simulink model "Control_Sim"  (R2023b)
settings: Solver=ode4  StartTime=0.0  StopTime=tf  FixedStep=tstep  RelTol=1e-3  EnableMultiTasking=on
values from neighbouring files (symbols this model uses):
  A_ref = [0 1;          -2*zeta*w_n_p -w_n_p^2]    [Velocity_Control.m]
  B_ref = [0; 1]    [Velocity_Control.m]
  count_map = zeros(length(theta),length(phi))    [Velocity_Control.m]
  g = 9.8065    [Velocity_Control.m]
  gamma_r = 0.05    [Velocity_Control.m]
  gamma_w = 0.1    [Velocity_Control.m]
  gamma_x = 1.*eye(2)    [Velocity_Control.m]
  I = diag([Ixx Iyy Izz])    [Velocity_Control.m]
  K_attitude = [10 2 0.2]    [Velocity_Control.m]
  K_orientation = zeros(3,6,length(phi)*length(theta))    [Velocity_Control.m]
  m = 1.5    [Velocity_Control.m]
  P_des = [0;0;5]    [Velocity_Control.m]
  P_lyap = lyap(A_ref, Q)    [Velocity_Control.m]
  tstep = 0.001    [Velocity_Control.m]
  wn_T = 0.1    [Velocity_Control.m]
libraries: simulink x1
settings Model: Creator=Nathan Dablain  LastModifiedBy=Nathan Dablain

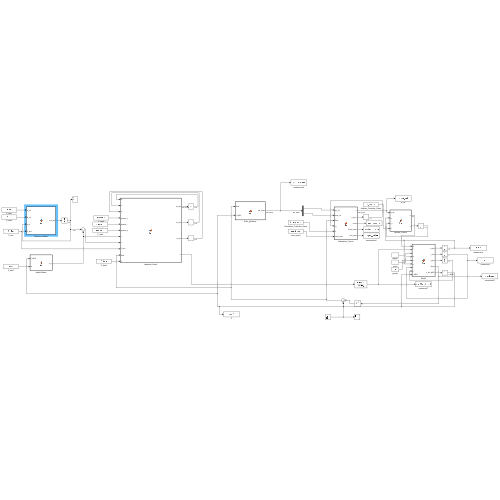
[thumbnail: Simulink's stored preview of the top-level diagram]
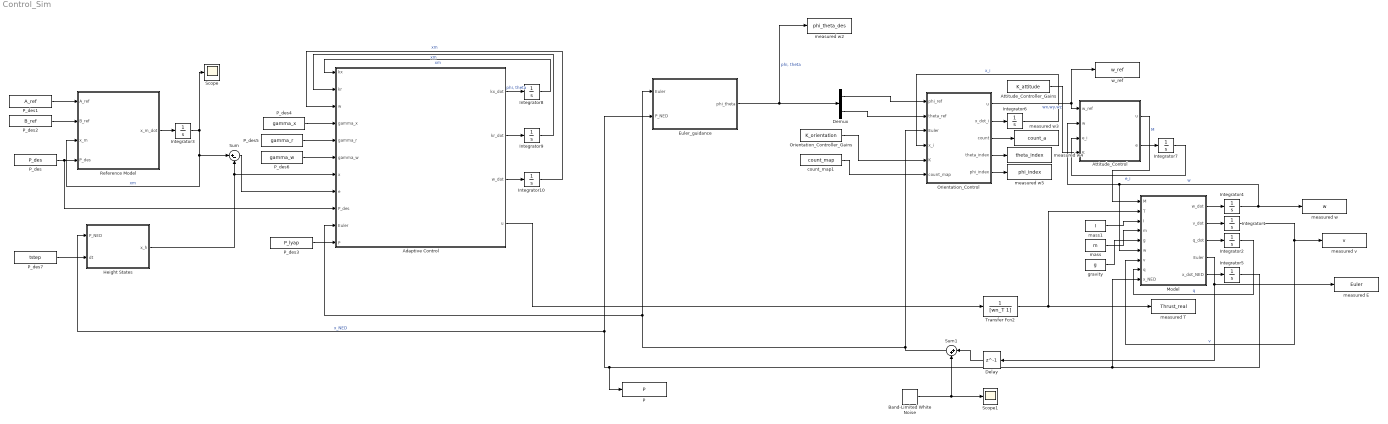
== system Control_Sim ==
  Adaptive Control : MATLAB Function  TreatAsAtomicUnit=on
  Attitude_Control : MATLAB Function  TreatAsAtomicUnit=on
  Attitude_Controller_Gains : Constant  Value=K_attitude
  Band-Limited White Noise : simulink/Sources/Band-Limited White Noise  Cov=[0.1; 0.1; 0.1].*1e-5  Ts=tstep  seed=[23341]
  Delay : Delay  DelayLength=1  InitialCondition=zeros(3,1)
  Demux : Demux  Outputs=2
  Euler_guidance : MATLAB Function  TreatAsAtomicUnit=on
  Height States : MATLAB Function  TreatAsAtomicUnit=on
  Integrator{1,4..7} (5 alike) : Integrator  InitialCondition=zeros(3,1)
  Integrator10 : Integrator
  Integrator2 : Integrator  InitialCondition=[1;0;0;0]
  Integrator3 : Integrator  InitialCondition=zeros(2,1)
  Integrator8 : Integrator  InitialCondition=zeros(2,1)
  Integrator9 : Integrator
  Model : MATLAB Function  TreatAsAtomicUnit=on
  Orientation_Control : MATLAB Function  TreatAsAtomicUnit=on
  Orientation_Controller_Gains : Constant  Value=K_orientation
  P : ToWorkspace  VariableName=P  SaveFormat=Structure  SampleTime=-1
  P_des : Constant  Value=P_des
  P_des1 : Constant  Value=A_ref
  P_des2 : Constant  Value=B_ref
  P_des3 : Constant  Value=P_lyap
  P_des4 : Constant  Value=gamma_x
  P_des5 : Constant  Value=gamma_r
  P_des6 : Constant  Value=gamma_w
  P_des7 : Constant  Value=tstep
  Reference Model : MATLAB Function  TreatAsAtomicUnit=on
  Scope : Scope
  Scope1 : Scope
  Sum : Sum  Inputs=|+-
  Sum1 : Sum  Inputs=|++
  Transfer Fcn2 : TransferFcn  Numerator=1  Denominator=[wn_T 1]
  count_map1 : Constant  Value=count_map
  gravity : Constant  Value=g
  mass : Constant  Value=m
  mass1 : Constant  Value=I
  measured E : ToWorkspace  VariableName=Euler  SaveFormat=Structure  SampleTime=-1
  measured T : ToWorkspace  VariableName=Thrust_real  SaveFormat=Structure  SampleTime=-1
  measured v : ToWorkspace  VariableName=v  SaveFormat=Structure  SampleTime=-1
  measured w : ToWorkspace  VariableName=w  SaveFormat=Structure  SampleTime=-1
  measured w2 : ToWorkspace  VariableName=phi_theta_des  SaveFormat=Structure  SampleTime=-1
  measured w3 : ToWorkspace  VariableName=count_a  SaveFormat=Structure  SampleTime=-1
  measured w4 : ToWorkspace  VariableName=theta_index  SaveFormat=Structure  SampleTime=-1
  measured w5 : ToWorkspace  VariableName=phi_index  SaveFormat=Structure  SampleTime=-1
  w_ref : ToWorkspace  VariableName=w_ref  SaveFormat=Structure  SampleTime=-1
  wires:
  gravity/1 -> Model/5(g)
  Integrator1/1 -> Model/7(v), measured v/1  "v"
  Model/2(v_dot) -> Integrator1/1
  mass/1 -> Model/4(m)
  Euler_guidance/1(phi_theta) -> measured w2/1, Demux/1  "phi, theta"
  Adaptive Control/4(u) -> Transfer Fcn2/1
  Transfer Fcn2/1 -> Model/2(T), measured T/1
  Model/4(Euler) -> measured E/1, Delay/1
  Model/3(q_dot) -> Integrator2/1
  Model/1(w_dot) -> Integrator4/1
  Integrator4/1 -> measured w/1, Attitude_Control/2(w), Model/6(w)  "w"
  Integrator2/1 -> Model/8(q)  "q"
  mass1/1 -> Model/3(I)
  Model/5(x_dot_NED) -> Integrator5/1
  Integrator5/1 -> Model/9(x_NED), Height States/1(P_NED), Euler_guidance/2(P_NED), P/1  "x_NED"
  Orientation_Control/2(x_dot_i) -> Integrator6/1
  Integrator6/1 -> Orientation_Control/4(x_i)  "x_i"
  Demux/1 -> Orientation_Control/1(phi_ref)
  Demux/2 -> Orientation_Control/2(theta_ref)
  Orientation_Controller_Gains/1 -> Orientation_Control/5(K)
  count_map1/1 -> Orientation_Control/6(count_map)
  Orientation_Control/1(u) -> Attitude_Control/1(w_ref), w_ref/1  "wx,wy,wz"
  Orientation_Control/3(count) -> measured w3/1
  Attitude_Control/2(e) -> Integrator7/1
  Integrator7/1 -> Attitude_Control/3(e_i)  "e_i"
  Attitude_Controller_Gains/1 -> Attitude_Control/4(K)
  Attitude_Control/1(u) -> Model/1(M)  "M"
  Orientation_Control/4(theta_index) -> measured w4/1
  Orientation_Control/5(phi_index) -> measured w5/1
  P_des/1 -> Adaptive Control/9(P_des), Reference Model/4(P_des)
  Integrator3/1 -> Scope/1, Sum/1, Reference Model/3(x_m)  "xm"
  Reference Model/1(x_m_dot) -> Integrator3/1
  P_des1/1 -> Reference Model/1(A_ref)
  P_des2/1 -> Reference Model/2(B_ref)
  Height States/1(x_h) -> Adaptive Control/7(x), Sum/2
  Adaptive Control/3(w_dot) -> Integrator10/1
  Adaptive Control/2(kr_dot) -> Integrator9/1
  Adaptive Control/1(kx_dot) -> Integrator8/1  "phi, theta"
  Integrator8/1 -> Adaptive Control/1(kx)  "xm"
  Integrator9/1 -> Adaptive Control/2(kr)  "xm"
  Integrator10/1 -> Adaptive Control/3(w)  "xm"
  Sum/1 -> Adaptive Control/8(e)
  P_des3/1 -> Adaptive Control/11(P)
  P_des4/1 -> Adaptive Control/4(gamma_x)
  P_des5/1 -> Adaptive Control/5(gamma_r)
  P_des6/1 -> Adaptive Control/6(gamma_w)
  P_des7/1 -> Height States/2(dt)
  Band-Limited White Noise/1 -> Scope1/1, Sum1/2
  Sum1/1 -> Adaptive Control/10(Euler), Euler_guidance/1(Euler), Orientation_Control/3(Euler)
  Delay/1 -> Sum1/1

== matlab function Control_Sim/Height States ==
  settings: updateMethod=DISCRETE
  data: x_h output; P_NED input; dt input
function x_h = fcn(P_NED, dt)
    persistent h_last;

    h = -1*P_NED(3);
    if isempty(h_last)
        h_last = h;
    end
    h_dot = (h - h_last)/dt;
    x_h = [h;h_dot];
    h_last = h;
end

== matlab function Control_Sim/Adaptive Control ==
  settings: updateMethod=DISCRETE
  data: kx input; kr input; w input; gamma_x input; gamma_r input; gamma_w input; x input; e input; P_des input; kx_dot output; Euler input; kr_dot output; w_dot output; u output; P input
function [kx_dot, kr_dot, w_dot, u] = fcn(kx, kr, w, gamma_x, gamma_r, gamma_w, x, e, P_des, Euler, P)
    % kx : 2x2 * 2x1 * 1x2 * 2x2 * 2x1 -> 2x1
    % kr : 1x1 * 1x1 * 1x2 * 2x2 * 2x1 -> 1x1
    % w : 1x1 * 1x1 * 1x2 * 2x2 * 2x1 -> 1x1
    B = [0;1];
    r = P_des(3);
    phi_x = cos(Euler(1))*cos(Euler(2));
    kx_dot = gamma_x*x*e'*P*B;
    kr_dot = gamma_r*r*e'*P*B;
    w_dot = gamma_w*phi_x*e'*P*B;
    
    u = kx'*x + kr*r - w'*phi_x;
    if u > 30; u = 30; end
    if u < 0; u = 0; end
end

== matlab function Control_Sim/Reference Model ==
  settings: updateMethod=DISCRETE
  data: x_m_dot output; A_ref input; B_ref input; x_m input; P_des input
function x_m_dot = fcn(A_ref, B_ref, x_m, P_des)
    r = P_des(3);
    x_m_dot = A_ref*x_m + B_ref*r;
end

== matlab function Control_Sim/Orientation_Control ==
  settings: updateMethod=DISCRETE
  data: u output; x_dot_i output; phi_ref input; theta_ref input; Euler input; x_i input; K input; count output; count_map input; theta_index output; phi_index output
function [u, x_dot_i, count, theta_index, phi_index] = fcn(phi_ref, theta_ref, Euler, x_i, K, count_map)
    phi_m = Euler(1)*180/pi;
    theta_m = Euler(2)*180/pi;
    theta = -20:5:20;
    phi = -20:5:20;
    theta_index = 1;
    phi_index = 1;
    for i = 1:length(theta)
        if abs(theta_m-theta(i)) <= 2.5
            theta_index = i;
            break;
        end
    end
    for i = 1:length(phi)
        if abs(phi_m-phi(i)) <= 2.5
            phi_index = i;
            break;
        end
    end
    count = count_map(theta_index,phi_index);
    Euler_des = [phi_ref;theta_ref;0];
    x_dot_i = Euler_des - Euler;
    x = [Euler; x_i];
    u = -K(:,:,count)*x;
end

== matlab function Control_Sim/Euler_guidance ==
  settings: updateMethod=DISCRETE
  data: phi_theta output; Euler input; P_NED input
function phi_theta = fcn(Euler, P_NED)
    % Want to map e_P_NED to Euler angles, psi is constrained to 0 by
    % default
    phi_theta = zeros(2,1);
end

== matlab function Control_Sim/Model ==
  data: w_dot output; M input; T input; I input; m input; g input; v_dot output; w input; v input; q input; q_dot output; Euler output; x_dot_NED output; x_NED input
function [w_dot, v_dot, q_dot, Euler, x_dot_NED] = fcn(M, T, I, m, g, w, v, q, x_NED)
    phi = atan2(2*(q(1)*q(2) + q(3)*q(4)),1-2*(q(2)^2+q(3)^2));
    theta = asin(2*(q(1)*q(3)-q(2)*q(4)));
    psi = atan2(2*(q(1)*q(4)+q(2)*q(3)), 1-2*(q(3)^2+q(4)^2));

    u = -1.*q(2:4);
    t = 2*cross(u, v);
    x_dot_NED = v + q(1)*t + cross(u, t);

    Euler = [phi;theta;psi];
    
    F_ground = 0;
    if x_NED(3) > 0
        ground_damping = 100;
        ground_stiffness = 1000;
        F_ground = ground_damping*x_dot_NED(3) + ground_stiffness*x_NED(3);
    end
    F = [(-m*g + F_ground)*sin(theta);...
         (m*g - F_ground)*sin(phi)*cos(theta);...
         (m*g - F_ground)*cos(phi)*cos(theta) - T];
    v_dot = F./m - cross(w,v);

    w_dot = I\(M - cross(w,I*w));

    omega = 0.5.*[0      -w(1)    -w(2)    -w(3);...
             w(1)  0       w(3)     -w(2);...
             w(2)  -w(3)   0       w(1);...
             w(3)  w(2)    -w(1)   0];
    q_dot = (omega*q)+(0.5*(1-dot(q,q))*q);
   
end

== matlab function Control_Sim/Attitude_Control ==
  settings: updateMethod=DISCRETE
  data: u output; e output; w_ref input; w input; e_i input; K input
function [u, e] = fcn(w_ref, w, e_i, K)
    persistent e_last;
    if isempty(e_last)
        e_last = zeros(3,1);
    end
    e = w_ref - w;
    e_d = e - e_last;
    u = zeros(3,1);
    for i = 1:3
        u(i) = K(1)*e(i) + K(2)*e_i(i) + K(3)*e_d(i);
    end
    e_last = e;
end
